simulink model "EXERCICE1"  (R2022b)
settings: Solver=VariableStepAuto  StartTime=0.0  StopTime=5  RelTol=1e-3
values from neighbouring files (symbols this model uses):
  A = [0, 1, 0, 0 ... (first row only)    [matrix.m]
  B = [0 ... (first row only)    [matrix.m]
  C = [1, 0, 0, 0 ... (first row only)    [matrix.m]
  K = lqr(A, B, R, Q, zeros)    [matrix.m]
  L = place(A', C', P)'    [matrix.m]
settings Model: Creator=mathe  LastModifiedBy=mathe

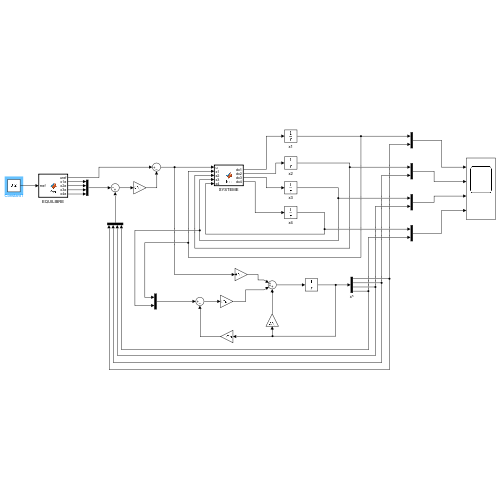
[thumbnail: Simulink's stored preview of the top-level diagram]
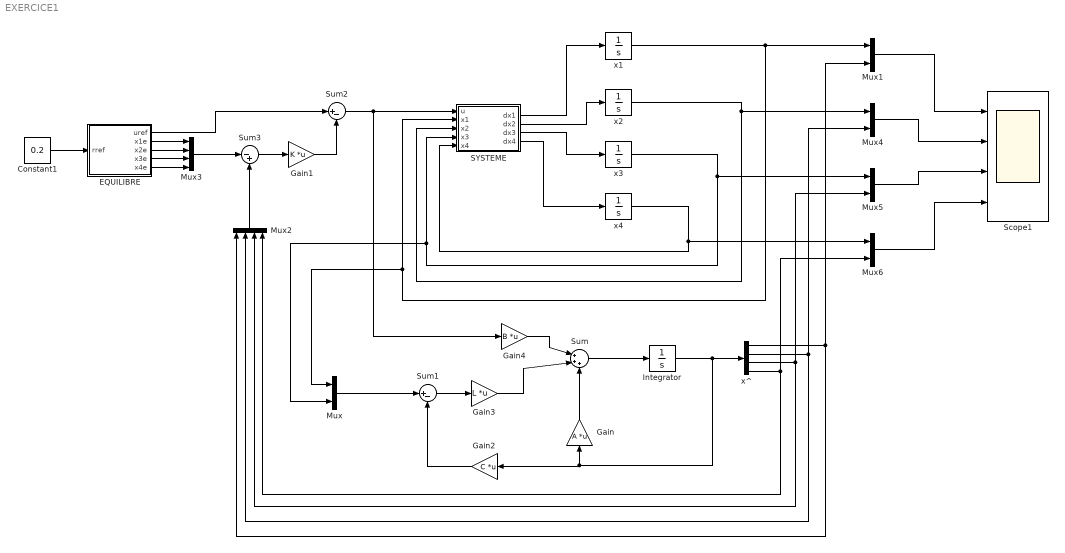
== system EXERCICE1 ==
  Constant1 : Constant  Value=0.2
  EQUILIBRE : MATLAB Function  TreatAsAtomicUnit=on
  Gain : Gain  Gain=A  Multiplication=Matrix(K*u)
  Gain1 : Gain  Gain=K  Multiplication=Matrix(K*u)
  Gain2 : Gain  Gain=C  Multiplication=Matrix(K*u)
  Gain3 : Gain  Gain=L  Multiplication=Matrix(K*u)
  Gain4 : Gain  Gain=B  Multiplication=Matrix(K*u)
  Integrator : Integrator
  Mux{,1,4..6} (5 alike) : Mux  Inputs=2
  Mux2 : Mux
  Mux3 : Mux
  SYSTEME : MATLAB Function  TreatAsAtomicUnit=on
  Scope1 : Scope  NumInputPorts=4
  Sum : Sum  Inputs=|+++
  Sum1 : Sum  Inputs=|+-
  Sum2 : Sum  Inputs=|+-
  Sum3 : Sum  Inputs=|-+
  x1 : Integrator  InitialCondition=0.1
  x2 : Integrator  InitialCondition=0.1
  x3 : Integrator
  x4 : Integrator
  x^ : Demux
  wires:
  SYSTEME/1(dx1) -> x1/1
  SYSTEME/2(dx2) -> x2/1
  SYSTEME/3(dx3) -> x3/1
  SYSTEME/4(dx4) -> x4/1
  x3/1 -> SYSTEME/4(x3), Mux/2, Mux5/1
  x4/1 -> SYSTEME/5(x4), Mux6/1
  Constant1/1 -> EQUILIBRE/1(rref)
  EQUILIBRE/3(x2e) -> Mux3/2
  Mux3/1 -> Sum3/1
  x2/1 -> SYSTEME/3(x2), Mux4/1
  x1/1 -> Mux1/1, SYSTEME/2(x1), Mux/1
  EQUILIBRE/4(x3e) -> Mux3/3
  EQUILIBRE/1(uref) -> Sum2/1
  Sum3/1 -> Gain1/1
  Gain1/1 -> Sum2/2
  EQUILIBRE/2(x1e) -> Mux3/1
  EQUILIBRE/5(x4e) -> Mux3/4
  Sum2/1 -> Gain4/1, SYSTEME/1(u)
  Sum/1 -> Integrator/1
  Sum1/1 -> Gain3/1
  Gain2/1 -> Sum1/2
  Gain/1 -> Sum/3
  Integrator/1 -> Gain2/1, Gain/1, x^/1
  Gain3/1 -> Sum/2
  Gain4/1 -> Sum/1
  Mux1/1 -> Scope1/1
  Mux4/1 -> Scope1/2
  x^/2 -> Mux2/2, Mux4/2
  Mux5/1 -> Scope1/3
  x^/3 -> Mux2/3, Mux5/2
  Mux6/1 -> Scope1/4
  x^/4 -> Mux6/2, Mux2/4
  Mux2/1 -> Sum3/2
  x^/1 -> Mux1/2, Mux2/1
  Mux/1 -> Sum1/1

== matlab function EXERCICE1/EQUILIBRE ==
  data: rref input; uref output; x1e output; x2e output; x3e output; x4e output
function [uref, x1e, x2e, x3e, x4e]  = fcn(rref)

%paramètres du système
m = 0.6;
g = 9.81;

%l'état d'équilibre
x1e = rref;
x2e = 0;
x3e = 0;
x4e = 0;

%commande d'équilibre
uref = m*g*rref;

== matlab function EXERCICE1/SYSTEME ==
  data: u input; x1 input; dx1 output; x2 input; dx2 output; x3 input; x4 input; dx3 output; dx4 output
function [dx1, dx2, dx3, dx4] = fcn(u, x1, x2, x3, x4)

%paramètres du système
J = 0.02;
m = 0.6;
sigma = 0.8;
g = 9.81;

%dynamique du système
dx1 = x2;
dx2 = (x1*(x4)^2 - g*sin(x3))/(1+sigma);
dx3 = x4;
dx4 = (u-m*g*x1*cos(x3)-2*m*x1*x2*x4)/(J+m*(x1)^2);
